simulink model "SW"  (R2016a)
settings: Solver=VariableStepAuto  StartTime=0.0  StopTime=10.0  RelTol=1e-3
undefined symbols (not defined in the file or in its folder): T
settings Model: Creator=gdlau  LastModifiedBy=gdlau

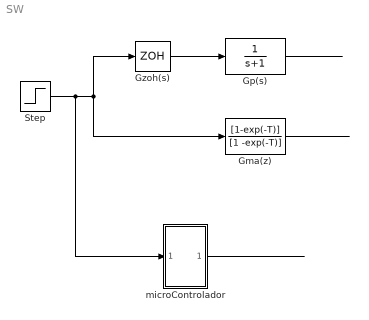
== system SW ==
  Gma(z) : DiscreteTransferFcn  Numerator=[1-exp(-T)]  Denominator=[1 -exp(-T)]
  Gp(s) : TransferFcn  Denominator=[1 1]
  Gzoh(s) : ZeroOrderHold
  Step : Step  SampleTime=0
  microControlador : Subsystem
  wires:
  Gzoh(s)/1 -> Gp(s)/1
  Step/1 -> microControlador/1(u(t)), Gzoh(s)/1, Gma(z)/1
  Gma(z)/1 -> ?
  Gp(s)/1 -> ?
  microControlador/1(Out1) -> ?

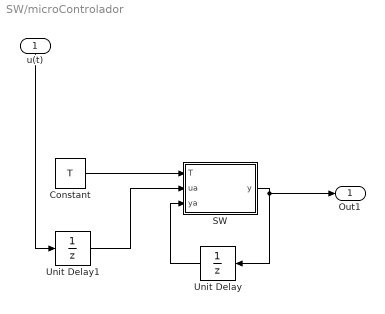
== system SW/microControlador ==
  u(t) : Inport
  Constant : Constant  Value=T
  SW : MATLAB Function  TreatAsAtomicUnit=on
  Unit Delay : UnitDelay  SampleTime=-1
  Unit Delay1 : UnitDelay  SampleTime=-1
  Out1 : Outport
  wires:
  u(t)/1 -> Unit Delay1/1
  Unit Delay1/1 -> SW/2(ua)
  Constant/1 -> SW/1(T)
  Unit Delay/1 -> SW/3(ya)
  SW/1(y) -> Out1/1, Unit Delay/1

== matlab function SW/microControlador/SW ==
  data: T input; y output; ua input; ya input
function y = ModeloSW(T, ua, ya)

%#codegen
a = 1-exp(-T)
b = exp(-T)
y = a*ua + b*ya;
